simulink model "nn_fuel_control_6_20"  (R2021a)
settings: Solver=ode15s  StartTime=0.0  StopTime=T  MaxStep=.01  RelTol=1e-3
undefined symbols (not defined in the file): AF_sensor_tol, fault_time, fuel_inj_tol, kappa_tol, MAF_sensor_tol, pump_tol, tau_ww_tol
libraries: neural x128
(part 2 of 6)

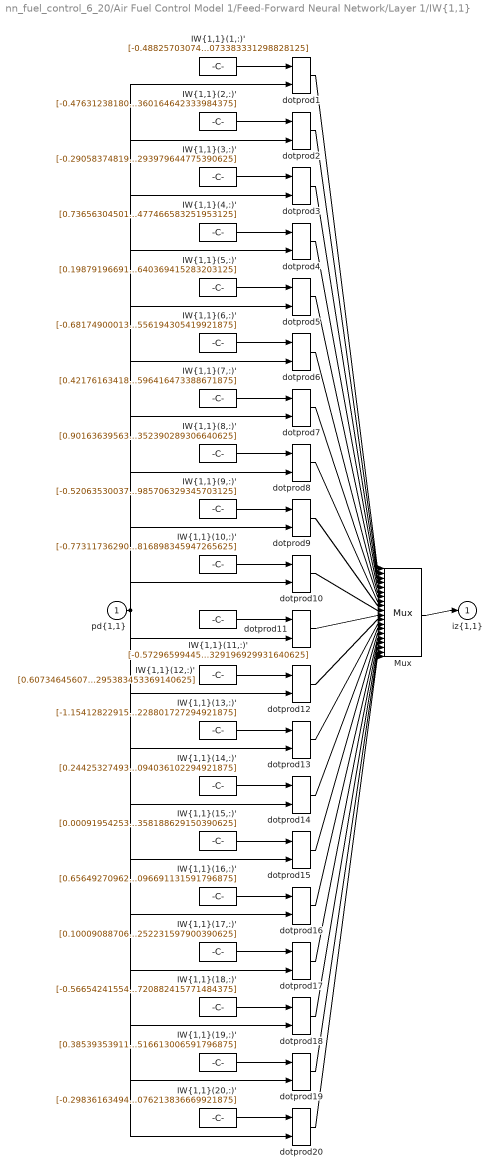
== system nn_fuel_control_6_20/Air Fuel Control Model 1/Feed-Forward Neural Network/Layer 1/IW{1,1} ==
  "pd{1,1}" : Inport  PortDimensions=4
      mask Display: e = 0.06;c1 = [120 230 180]/255;c2 = ([120 230 180]+0)/(256+128);c3 = ([120 230 180]+128)/(256+128);patch([0 1 1 0],[0 0 1 1],c1);patch([0 1 1 1-e 1-e 0+e],[0 0 1 1-e 0+e 0+e],c2);patch([0 0 1 1-e 0+e 0+e],[0 1 1 1-e 1-e 0+e],c3);plot([0 1 1 0 0],[0 0 1 1 0]);
  "IW{1,1}(1,:)'" : Constant  Value=[-0.48825703074007853476956597660318948328495025634765625;-0.571856754184941085128457416431047022342681884765625;-0.40434581347511555637908031712868250906467437744140625;0.33801748115781393710932434260030277073383331298828125]
      mask Display: e = 0.06;c1 = [120 150 230]/255;c2 = ([120 150 230]+0)/383;c3 = ([120 150 230]+128)/383;patch([0 1 1 0],[0 0 1 1],c1);patch([0 1 1 1-e 1-e 0+e],[0 0 1 1-e 0+e 0+e],c2);patch([0 0 1 1-e 0+e 0+e],[0 1 1 1-e 1-e 0+e],c3);plot([0 1 1 0 0],[0 0 1 1 0]);disp('Weights');
  "IW{1,1}(10,:)'" : Constant  Value=[-0.7731173629085674736671762730111368000507354736328125;0.2005059506174451389171053961035795509815216064453125;0.1626130441440647445006106863729655742645263671875;0.1745533013814315470568772070691920816898345947265625]
      mask Display: e = 0.06;c1 = [120 150 230]/255;c2 = ([120 150 230]+0)/383;c3 = ([120 150 230]+128)/383;patch([0 1 1 0],[0 0 1 1],c1);patch([0 1 1 1-e 1-e 0+e],[0 0 1 1-e 0+e 0+e],c2);patch([0 0 1 1-e 0+e 0+e],[0 1 1 1-e 1-e 0+e],c3);plot([0 1 1 0 0],[0 0 1 1 0]);disp('Weights');
  "IW{1,1}(11,:)'" : Constant  Value=[-0.57296599445932028249472978131962008774280548095703125;0.486466690002032298156819933865335769951343536376953125;0.59005984322004934039540557932923547923564910888671875;0.478764443667865580156473015449591912329196929931640625]
      mask Display: e = 0.06;c1 = [120 150 230]/255;c2 = ([120 150 230]+0)/383;c3 = ([120 150 230]+128)/383;patch([0 1 1 0],[0 0 1 1],c1);patch([0 1 1 1-e 1-e 0+e],[0 0 1 1-e 0+e 0+e],c2);patch([0 0 1 1-e 0+e 0+e],[0 1 1 1-e 1-e 0+e],c3);plot([0 1 1 0 0],[0 0 1 1 0]);disp('Weights');
  "IW{1,1}(12,:)'" : Constant  Value=[0.60734645607013415524733090933295898139476776123046875;-0.56727561458132924609998326559434644877910614013671875;-0.3464328462213754900034246020368300378322601318359375;0.01188492491926852225037070098778713145293295383453369140625]
      mask Display: e = 0.06;c1 = [120 150 230]/255;c2 = ([120 150 230]+0)/383;c3 = ([120 150 230]+128)/383;patch([0 1 1 0],[0 0 1 1],c1);patch([0 1 1 1-e 1-e 0+e],[0 0 1 1-e 0+e 0+e],c2);patch([0 0 1 1-e 0+e 0+e],[0 1 1 1-e 1-e 0+e],c3);plot([0 1 1 0 0],[0 0 1 1 0]);disp('Weights');
  "IW{1,1}(13,:)'" : Constant  Value=[-1.1541282291561423267722830132697708904743194580078125;-0.367041931636175267072985661798156797885894775390625;0.00571687256956400491336722780033596791326999664306640625;-1.1769488295019250312378744638408534228801727294921875]
      mask Display: e = 0.06;c1 = [120 150 230]/255;c2 = ([120 150 230]+0)/383;c3 = ([120 150 230]+128)/383;patch([0 1 1 0],[0 0 1 1],c1);patch([0 1 1 1-e 1-e 0+e],[0 0 1 1-e 0+e 0+e],c2);patch([0 0 1 1-e 0+e 0+e],[0 1 1 1-e 1-e 0+e],c3);plot([0 1 1 0 0],[0 0 1 1 0]);disp('Weights');
  "IW{1,1}(14,:)'" : Constant  Value=[0.2442532749352764043226926560237188823521137237548828125;-1.8079559641845570627793904350255616009235382080078125;-0.84702514936941530887537510352558456361293792724609375;0.71981418547994457934890988326515071094036102294921875]
      mask Display: e = 0.06;c1 = [120 150 230]/255;c2 = ([120 150 230]+0)/383;c3 = ([120 150 230]+128)/383;patch([0 1 1 0],[0 0 1 1],c1);patch([0 1 1 1-e 1-e 0+e],[0 0 1 1-e 0+e 0+e],c2);patch([0 0 1 1-e 0+e 0+e],[0 1 1 1-e 1-e 0+e],c3);plot([0 1 1 0 0],[0 0 1 1 0]);disp('Weights');
  "IW{1,1}(15,:)'" : Constant  Value=[0.00091954253676776779267976191789557560696266591548919677734375;0.58230594094139209726535000299918465316295623779296875;-0.1812579368778876320877913030926720239222049713134765625;0.81865583686941756358379507219069637358188629150390625]
      mask Display: e = 0.06;c1 = [120 150 230]/255;c2 = ([120 150 230]+0)/383;c3 = ([120 150 230]+128)/383;patch([0 1 1 0],[0 0 1 1],c1);patch([0 1 1 1-e 1-e 0+e],[0 0 1 1-e 0+e 0+e],c2);patch([0 0 1 1-e 0+e 0+e],[0 1 1 1-e 1-e 0+e],c3);plot([0 1 1 0 0],[0 0 1 1 0]);disp('Weights');
  "IW{1,1}(16,:)'" : Constant  Value=[0.65649270962487193958878606281359679996967315673828125;-0.76315614470481663023093688025255687534809112548828125;0.301942106699343681963654262290219776332378387451171875;0.17120717116793560119702988231438212096691131591796875]
      mask Display: e = 0.06;c1 = [120 150 230]/255;c2 = ([120 150 230]+0)/383;c3 = ([120 150 230]+128)/383;patch([0 1 1 0],[0 0 1 1],c1);patch([0 1 1 1-e 1-e 0+e],[0 0 1 1-e 0+e 0+e],c2);patch([0 0 1 1-e 0+e 0+e],[0 1 1 1-e 1-e 0+e],c3);plot([0 1 1 0 0],[0 0 1 1 0]);disp('Weights');
  "IW{1,1}(17,:)'" : Constant  Value=[0.10009088706659761969230970635180710814893245697021484375;0.283349138687722490459464097511954605579376220703125;-0.33980594650471385165246829274110496044158935546875;0.0191029179120060545182813172004898660816252231597900390625]
      mask Display: e = 0.06;c1 = [120 150 230]/255;c2 = ([120 150 230]+0)/383;c3 = ([120 150 230]+128)/383;patch([0 1 1 0],[0 0 1 1],c1);patch([0 1 1 1-e 1-e 0+e],[0 0 1 1-e 0+e 0+e],c2);patch([0 0 1 1-e 0+e 0+e],[0 1 1 1-e 1-e 0+e],c3);plot([0 1 1 0 0],[0 0 1 1 0]);disp('Weights');
  "IW{1,1}(18,:)'" : Constant  Value=[-0.5665424155432698949397263277205638587474822998046875;-0.54033955185199145088148497961810790002346038818359375;0.279081720790874066029374489517067559063434600830078125;0.47911903792710874849802848984836600720882415771484375]
      mask Display: e = 0.06;c1 = [120 150 230]/255;c2 = ([120 150 230]+0)/383;c3 = ([120 150 230]+128)/383;patch([0 1 1 0],[0 0 1 1],c1);patch([0 1 1 1-e 1-e 0+e],[0 0 1 1-e 0+e 0+e],c2);patch([0 0 1 1-e 0+e 0+e],[0 1 1 1-e 1-e 0+e],c3);plot([0 1 1 0 0],[0 0 1 1 0]);disp('Weights');
  "IW{1,1}(19,:)'" : Constant  Value=[0.3853935391181619873890440430841408669948577880859375;-0.383574085589689861564011152950115501880645751953125;-0.5416431443522891076014502687030471861362457275390625;-0.981747569426136390546844268101267516613006591796875]
      mask Display: e = 0.06;c1 = [120 150 230]/255;c2 = ([120 150 230]+0)/383;c3 = ([120 150 230]+128)/383;patch([0 1 1 0],[0 0 1 1],c1);patch([0 1 1 1-e 1-e 0+e],[0 0 1 1-e 0+e 0+e],c2);patch([0 0 1 1-e 0+e 0+e],[0 1 1 1-e 1-e 0+e],c3);plot([0 1 1 0 0],[0 0 1 1 0]);disp('Weights');
  "IW{1,1}(2,:)'" : Constant  Value=[-0.4763123818029502132276320480741560459136962890625;-0.3624779463226779352424955504829995334148406982421875;0.548920167863276020625562523491680622100830078125;-0.9809602571508406754219322465360164642333984375]
      mask Display: e = 0.06;c1 = [120 150 230]/255;c2 = ([120 150 230]+0)/383;c3 = ([120 150 230]+128)/383;patch([0 1 1 0],[0 0 1 1],c1);patch([0 1 1 1-e 1-e 0+e],[0 0 1 1-e 0+e 0+e],c2);patch([0 0 1 1-e 0+e 0+e],[0 1 1 1-e 1-e 0+e],c3);plot([0 1 1 0 0],[0 0 1 1 0]);disp('Weights');
  "IW{1,1}(20,:)'" : Constant  Value=[-0.2983616349407973711294062013621442019939422607421875;-0.904882675555897630914614637731574475765228271484375;0.3663740946078786198114585204166360199451446533203125;-0.377532327383313326407687782193534076213836669921875]
      mask Display: e = 0.06;c1 = [120 150 230]/255;c2 = ([120 150 230]+0)/383;c3 = ([120 150 230]+128)/383;patch([0 1 1 0],[0 0 1 1],c1);patch([0 1 1 1-e 1-e 0+e],[0 0 1 1-e 0+e 0+e],c2);patch([0 0 1 1-e 0+e 0+e],[0 1 1 1-e 1-e 0+e],c3);plot([0 1 1 0 0],[0 0 1 1 0]);disp('Weights');
  "IW{1,1}(3,:)'" : Constant  Value=[-0.2905837481960433787975262021063826978206634521484375;0.109981844822967911312616706709377467632293701171875;0.455515839932046084914674111132626421749591827392578125;-0.8132927338045536913568867021240293979644775390625]
      mask Display: e = 0.06;c1 = [120 150 230]/255;c2 = ([120 150 230]+0)/383;c3 = ([120 150 230]+128)/383;patch([0 1 1 0],[0 0 1 1],c1);patch([0 1 1 1-e 1-e 0+e],[0 0 1 1-e 0+e 0+e],c2);patch([0 0 1 1-e 0+e 0+e],[0 1 1 1-e 1-e 0+e],c3);plot([0 1 1 0 0],[0 0 1 1 0]);disp('Weights');
  "IW{1,1}(4,:)'" : Constant  Value=[0.73656304501564962006199266397743485867977142333984375;-3.144535832691242038805512493127025663852691650390625;-1.0375718682022092576033855948480777442455291748046875;0.64654475977152092713851061489549465477466583251953125]
      mask Display: e = 0.06;c1 = [120 150 230]/255;c2 = ([120 150 230]+0)/383;c3 = ([120 150 230]+128)/383;patch([0 1 1 0],[0 0 1 1],c1);patch([0 1 1 1-e 1-e 0+e],[0 0 1 1-e 0+e 0+e],c2);patch([0 0 1 1-e 0+e 0+e],[0 1 1 1-e 1-e 0+e],c3);plot([0 1 1 0 0],[0 0 1 1 0]);disp('Weights');
  "IW{1,1}(5,:)'" : Constant  Value=[0.198791966914059037296880205758498050272464752197265625;-0.1633450522665338133787571450739051215350627899169921875;0.42744201772333045852292343624867498874664306640625;0.256072707330624649291195282785338349640369415283203125]
      mask Display: e = 0.06;c1 = [120 150 230]/255;c2 = ([120 150 230]+0)/383;c3 = ([120 150 230]+128)/383;patch([0 1 1 0],[0 0 1 1],c1);patch([0 1 1 1-e 1-e 0+e],[0 0 1 1-e 0+e 0+e],c2);patch([0 0 1 1-e 0+e 0+e],[0 1 1 1-e 1-e 0+e],c3);plot([0 1 1 0 0],[0 0 1 1 0]);disp('Weights');
  "IW{1,1}(6,:)'" : Constant  Value=[-0.68174900013601558157461113296449184417724609375;-0.143660359213997057548084512745845131576061248779296875;-0.017244855890485570604209186740263248793780803680419921875;-0.59564977304797117607648715420509688556194305419921875]
      mask Display: e = 0.06;c1 = [120 150 230]/255;c2 = ([120 150 230]+0)/383;c3 = ([120 150 230]+128)/383;patch([0 1 1 0],[0 0 1 1],c1);patch([0 1 1 1-e 1-e 0+e],[0 0 1 1-e 0+e 0+e],c2);patch([0 0 1 1-e 0+e 0+e],[0 1 1 1-e 1-e 0+e],c3);plot([0 1 1 0 0],[0 0 1 1 0]);disp('Weights');
  "IW{1,1}(7,:)'" : Constant  Value=[0.4217616341804173440976910569588653743267059326171875;0.268686773032350334489137821947224438190460205078125;-0.7596642819355239328871221005101688206195831298828125;0.1140485715139589739663961154292337596416473388671875]
      mask Display: e = 0.06;c1 = [120 150 230]/255;c2 = ([120 150 230]+0)/383;c3 = ([120 150 230]+128)/383;patch([0 1 1 0],[0 0 1 1],c1);patch([0 1 1 1-e 1-e 0+e],[0 0 1 1-e 0+e 0+e],c2);patch([0 0 1 1-e 0+e 0+e],[0 1 1 1-e 1-e 0+e],c3);plot([0 1 1 0 0],[0 0 1 1 0]);disp('Weights');
  "IW{1,1}(8,:)'" : Constant  Value=[0.9016363956360040621262896820553578436374664306640625;0.357548177780251108526243797314236871898174285888671875;0.55252323002836389864711463815183378756046295166015625;-0.060258972495788688805706811990603455342352390289306640625]
      mask Display: e = 0.06;c1 = [120 150 230]/255;c2 = ([120 150 230]+0)/383;c3 = ([120 150 230]+128)/383;patch([0 1 1 0],[0 0 1 1],c1);patch([0 1 1 1-e 1-e 0+e],[0 0 1 1-e 0+e 0+e],c2);patch([0 0 1 1-e 0+e 0+e],[0 1 1 1-e 1-e 0+e],c3);plot([0 1 1 0 0],[0 0 1 1 0]);disp('Weights');
  "IW{1,1}(9,:)'" : Constant  Value=[-0.52063530037897998159479584501241333782672882080078125;0.81677809495395992112065641777007840573787689208984375;-0.95310858934972031430987726707826368510723114013671875;0.325348652875194599420893837304902262985706329345703125]
      mask Display: e = 0.06;c1 = [120 150 230]/255;c2 = ([120 150 230]+0)/383;c3 = ([120 150 230]+128)/383;patch([0 1 1 0],[0 0 1 1],c1);patch([0 1 1 1-e 1-e 0+e],[0 0 1 1-e 0+e 0+e],c2);patch([0 0 1 1-e 0+e 0+e],[0 1 1 1-e 1-e 0+e],c3);plot([0 1 1 0 0],[0 0 1 1 0]);disp('Weights');
  Mux : Mux  Inputs=20
      mask Display: e = 0.06;c1 = [120 150 230]/255;c2 = ([120 150 230]+0)/383;c3 = ([120 150 230]+128)/383;patch([0 1 1 0],[0 0 1 1],c1);patch([0 1 1 1-e 1-e 0+e],[0 0 1 1-e 0+e 0+e],c2);patch([0 0 1 1-e 0+e 0+e],[0 1 1 1-e 1-e 0+e],c3);plot([0 1 1 0 0],[0 0 1 1 0]);disp('Mux');
  dotprod{1..20} (20 alike) : neural/Weight Functions/dotprod
  "iz{1,1}" : Outport
      mask Display: e = 0.06;c1 = [120 230 180]/255;c2 = ([120 230 180]+0)/(256+128);c3 = ([120 230 180]+128)/(256+128);patch([0 1 1 0],[0 0 1 1],c1);patch([0 1 1 1-e 1-e 0+e],[0 0 1 1-e 0+e 0+e],c2);patch([0 0 1 1-e 0+e 0+e],[0 1 1 1-e 1-e 0+e],c3);plot([0 1 1 0 0],[0 0 1 1 0]);
  wires:
  "IW{1,1}(1,:)'"/1 -> dotprod1/1
  "pd{1,1}"/1 -> dotprod1/2, dotprod2/2, dotprod3/2, dotprod4/2, dotprod5/2, dotprod6/2, dotprod7/2, dotprod8/2, dotprod9/2, dotprod10/2, dotprod11/2, dotprod12/2, dotprod13/2, dotprod14/2, dotprod15/2, dotprod16/2, dotprod17/2, dotprod18/2, dotprod19/2, dotprod20/2
  dotprod1/1 -> Mux/1
  "IW{1,1}(2,:)'"/1 -> dotprod2/1
  dotprod2/1 -> Mux/2
  "IW{1,1}(3,:)'"/1 -> dotprod3/1
  dotprod3/1 -> Mux/3
  "IW{1,1}(4,:)'"/1 -> dotprod4/1
  dotprod4/1 -> Mux/4
  "IW{1,1}(5,:)'"/1 -> dotprod5/1
  dotprod5/1 -> Mux/5
  "IW{1,1}(6,:)'"/1 -> dotprod6/1
  dotprod6/1 -> Mux/6
  "IW{1,1}(7,:)'"/1 -> dotprod7/1
  dotprod7/1 -> Mux/7
  "IW{1,1}(8,:)'"/1 -> dotprod8/1
  dotprod8/1 -> Mux/8
  "IW{1,1}(9,:)'"/1 -> dotprod9/1
  dotprod9/1 -> Mux/9
  "IW{1,1}(10,:)'"/1 -> dotprod10/1
  dotprod10/1 -> Mux/10
  "IW{1,1}(11,:)'"/1 -> dotprod11/1
  dotprod11/1 -> Mux/11
  "IW{1,1}(12,:)'"/1 -> dotprod12/1
  dotprod12/1 -> Mux/12
  "IW{1,1}(13,:)'"/1 -> dotprod13/1
  dotprod13/1 -> Mux/13
  "IW{1,1}(14,:)'"/1 -> dotprod14/1
  dotprod14/1 -> Mux/14
  "IW{1,1}(15,:)'"/1 -> dotprod15/1
  dotprod15/1 -> Mux/15
  "IW{1,1}(16,:)'"/1 -> dotprod16/1
  dotprod16/1 -> Mux/16
  "IW{1,1}(17,:)'"/1 -> dotprod17/1
  dotprod17/1 -> Mux/17
  "IW{1,1}(18,:)'"/1 -> dotprod18/1
  dotprod18/1 -> Mux/18
  "IW{1,1}(19,:)'"/1 -> dotprod19/1
  dotprod19/1 -> Mux/19
  "IW{1,1}(20,:)'"/1 -> dotprod20/1
  dotprod20/1 -> Mux/20
  Mux/1 -> "iz{1,1}"/1

== system nn_fuel_control_6_20/Air Fuel Control Model 1/Feed-Forward Neural Network/Layer 2/Delays 1 ==
  "p{2}" : Inport  PortDimensions=20
      mask Display: e = 0.06;c1 = [120 230 180]/255;c2 = ([120 230 180]+0)/(256+128);c3 = ([120 230 180]+128)/(256+128);patch([0 1 1 0],[0 0 1 1],c1);patch([0 1 1 1-e 1-e 0+e],[0 0 1 1-e 0+e 0+e],c2);patch([0 0 1 1-e 0+e 0+e],[0 1 1 1-e 1-e 0+e],c3);plot([0 1 1 0 0],[0 0 1 1 0]);
  mux : Mux  Inputs=1
      mask Display: e = 0.06;c1 = [120 150 230]/255;c2 = ([120 150 230]+0)/383;c3 = ([120 150 230]+128)/383;patch([0 1 1 0],[0 0 1 1],c1);patch([0 1 1 1-e 1-e 0+e],[0 0 1 1-e 0+e 0+e],c2);patch([0 0 1 1-e 0+e 0+e],[0 1 1 1-e 1-e 0+e],c3);plot([0 1 1 0 0],[0 0 1 1 0]);disp('Mux')
  "pd{2,1}" : Outport
      mask Display: e = 0.06;c1 = [120 230 180]/255;c2 = ([120 230 180]+0)/(256+128);c3 = ([120 230 180]+128)/(256+128);patch([0 1 1 0],[0 0 1 1],c1);patch([0 1 1 1-e 1-e 0+e],[0 0 1 1-e 0+e 0+e],c2);patch([0 0 1 1-e 0+e 0+e],[0 1 1 1-e 1-e 0+e],c3);plot([0 1 1 0 0],[0 0 1 1 0]);
  wires:
  "p{2}"/1 -> mux/1
  mux/1 -> "pd{2,1}"/1

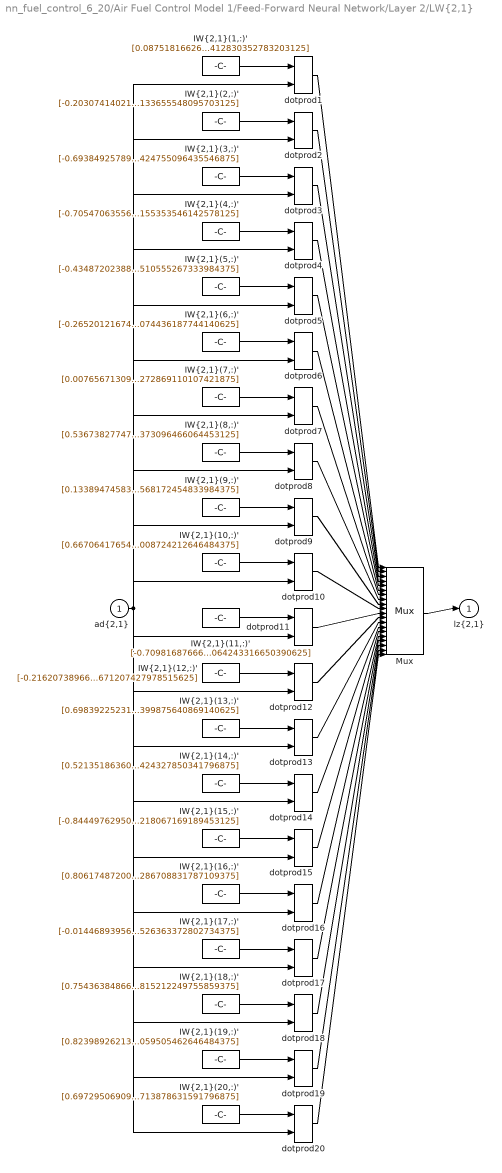
== system nn_fuel_control_6_20/Air Fuel Control Model 1/Feed-Forward Neural Network/Layer 2/LW{2,1} ==
  "ad{2,1}" : Inport  PortDimensions=20
      mask Display: e = 0.06;c1 = [120 230 180]/255;c2 = ([120 230 180]+0)/(256+128);c3 = ([120 230 180]+128)/(256+128);patch([0 1 1 0],[0 0 1 1],c1);patch([0 1 1 1-e 1-e 0+e],[0 0 1 1-e 0+e 0+e],c2);patch([0 0 1 1-e 0+e 0+e],[0 1 1 1-e 1-e 0+e],c3);plot([0 1 1 0 0],[0 0 1 1 0]);
  "IW{2,1}(1,:)'" : Constant  Value=[0.0875181662665719117821794270639657042920589447021484375;0.921321050546581421514247267623431980609893798828125;-0.1717118974253677432528775170794688165187835693359375;-0.68304825916014200171133552430546842515468597412109375;0.452339285545516556208411884654196910560131072998046875;-0.04529182730159657388480098916261340491473674774169921875;-0.9709510342483935740887091014883480966091156005859375;0.020509492560360172153099966863010195083916187286376953125;0.78509599817010677913486915713292546570301055908203125;-0.4830724448255014902287030054139904677867889404296875;0.89266777388446183483239337874692864716053009033203125;0.042941053928391655081231448320977506227791309356689453125;-0.1415144968584703122349566228876938112080097198486328125;-1.2230150910133141817226487546577118337154388427734375;0.1333293552699185424703642866006703115999698638916015625;-0.9177651014595056278011497852276079356670379638671875;-0.1228244578666999320404329409939236938953399658203125;0.5867901928731706906461340622627176344394683837890625;0.63198665556140465326961930259130895137786865234375;0.8997269280854862660845583377522416412830352783203125]
      mask Display: e = 0.06;c1 = [120 150 230]/255;c2 = ([120 150 230]+0)/383;c3 = ([120 150 230]+128)/383;patch([0 1 1 0],[0 0 1 1],c1);patch([0 1 1 1-e 1-e 0+e],[0 0 1 1-e 0+e 0+e],c2);patch([0 0 1 1-e 0+e 0+e],[0 1 1 1-e 1-e 0+e],c3);plot([0 1 1 0 0],[0 0 1 1 0]);disp('weights');
  "IW{2,1}(10,:)'" : Constant  Value=[0.6670641765450044946561547476449050009250640869140625;-0.514079267728301037010396612458862364292144775390625;0.4412099253120829178698159012128598988056182861328125;0.365585408566961145293561230573686771094799041748046875;-0.101844567281333564512380007727188058197498321533203125;1.0234943592269705181507788438466377556324005126953125;-0.2964378932206355177214618379366584122180938720703125;0.89165504879323720377470863240887410938739776611328125;0.00071741415381627871017400366326910443603992462158203125;-0.35129661907085729666277984506450593471527099609375;-0.08630387658328413091890496389169129543006420135498046875;0.73285931796011050121109065003111027181148529052734375;0.9141116517940217622850695988745428621768951416015625;-0.5898122749869834091640541373635642230510711669921875;0.5581383460192237411234827959560789167881011962890625;-0.391394620189690234379753519533551298081874847412109375;-0.56609108316777534408714700475684367120265960693359375;-0.78857350176913987294113894677138887345790863037109375;-0.1110936003246558723134285173728130757808685302734375;0.144677769719792959079995853244327008724212646484375]
      mask Display: e = 0.06;c1 = [120 150 230]/255;c2 = ([120 150 230]+0)/383;c3 = ([120 150 230]+128)/383;patch([0 1 1 0],[0 0 1 1],c1);patch([0 1 1 1-e 1-e 0+e],[0 0 1 1-e 0+e 0+e],c2);patch([0 0 1 1-e 0+e 0+e],[0 1 1 1-e 1-e 0+e],c3);plot([0 1 1 0 0],[0 0 1 1 0]);disp('weights');
  "IW{2,1}(11,:)'" : Constant  Value=[-0.709816876661096163303454886772669851779937744140625;-0.3444212300521931613417336848215200006961822509765625;0.9832500828514560975435188083793036639690399169921875;-0.43613745027057049252761089519481174647808074951171875;-0.55211644185470853951613889876171015202999114990234375;-0.7575041344288002687079597308184020221233367919921875;-0.2847945211821218958192503123427741229534149169921875;-0.07355592846682361407584238577328505925834178924560546875;0.634284151179720812052664768998511135578155517578125;-0.442299985847484311562993752886541187763214111328125;0.2745419011869854042373617630801163613796234130859375;-0.78469757805809281503428564974456094205379486083984375;-0.9078653485353538332702783009153790771961212158203125;0.08518212744205312658696271910230279900133609771728515625;-0.63299556814274715588197750548715703189373016357421875;0.94372659672676306730210171735961921513080596923828125;-0.86235896127647826414630571889574639499187469482421875;-0.36254626539261336493069620701135136187076568603515625;-0.9987256219878009044776945302146486937999725341796875;0.56472885556065310908024912350811064243316650390625]
      mask Display: e = 0.06;c1 = [120 150 230]/255;c2 = ([120 150 230]+0)/383;c3 = ([120 150 230]+128)/383;patch([0 1 1 0],[0 0 1 1],c1);patch([0 1 1 1-e 1-e 0+e],[0 0 1 1-e 0+e 0+e],c2);patch([0 0 1 1-e 0+e 0+e],[0 1 1 1-e 1-e 0+e],c3);plot([0 1 1 0 0],[0 0 1 1 0]);disp('weights');
  "IW{2,1}(12,:)'" : Constant  Value=[-0.2162073896661820260334252452594228088855743408203125;-0.761704303295197338030675382469780743122100830078125;0.124054668622003816391696773280273191630840301513671875;0.0666422255806751184792346975882537662982940673828125;-0.1018576594486159392349833296975702978670597076416015625;-0.7633396770781526452509524460765533149242401123046875;0.80878320521564450729101736214943230152130126953125;0.9107228523006707376907797879539430141448974609375;0.68803687900472876304291958149406127631664276123046875;-0.673404946456113151498357183299958705902099609375;0.02618620323267932537003588322477298788726329803466796875;-0.1434357633318594504867604655373725108802318572998046875;-0.2081794769619056684195612660914775915443897247314453125;0.82206885550436370468929681010195054113864898681640625;1.3395412792208656327375138062052428722381591796875;0.5779458927466978312992296196171082556247711181640625;-0.026880949945973141301802655789288110099732875823974609375;0.850129415928704279536987087340094149112701416015625;0.761799842289866635525186211452819406986236572265625;-0.7519111742583659552252584035159088671207427978515625]
      mask Display: e = 0.06;c1 = [120 150 230]/255;c2 = ([120 150 230]+0)/383;c3 = ([120 150 230]+128)/383;patch([0 1 1 0],[0 0 1 1],c1);patch([0 1 1 1-e 1-e 0+e],[0 0 1 1-e 0+e 0+e],c2);patch([0 0 1 1-e 0+e 0+e],[0 1 1 1-e 1-e 0+e],c3);plot([0 1 1 0 0],[0 0 1 1 0]);disp('weights');
  "IW{2,1}(13,:)'" : Constant  Value=[0.698392252312435513061927849776111543178558349609375;0.2006250289554845078754397036391310393810272216796875;0.8979808453752837760220018026302568614482879638671875;0.13058294946861292995521353077492676675319671630859375;0.6337289839007096414746911250404082238674163818359375;-0.4606636658097738035166912595741450786590576171875;0.58270529187201436371879026410169899463653564453125;-0.334455647345431150707639744723564945161342620849609375;0.432404381050130848240797831749659962952136993408203125;-0.5325686929910187217274142312817275524139404296875;-1.071395629971807039737541344948112964630126953125;0.01201015671242645910243851403720327652990818023681640625;-0.86364459893233791465405602139071561396121978759765625;0.44599042299617075446604985700105316936969757080078125;0.387361224848535135034666154751903377473354339599609375;0.5979970960929346102119552597287110984325408935546875;0.0432920224562478583862912273616530001163482666015625;0.347379189552733003143458745398675091564655303955078125;-0.810953983836439906696114121587015688419342041015625;0.123159835575779030847343165078200399875640869140625]
      mask Display: e = 0.06;c1 = [120 150 230]/255;c2 = ([120 150 230]+0)/383;c3 = ([120 150 230]+128)/383;patch([0 1 1 0],[0 0 1 1],c1);patch([0 1 1 1-e 1-e 0+e],[0 0 1 1-e 0+e 0+e],c2);patch([0 0 1 1-e 0+e 0+e],[0 1 1 1-e 1-e 0+e],c3);plot([0 1 1 0 0],[0 0 1 1 0]);disp('weights');
  "IW{2,1}(14,:)'" : Constant  Value=[0.52135186360587326692694887242396362125873565673828125;0.76681461221118496496274019591510295867919921875;0.182440316929996904082855735396151430904865264892578125;-0.667185236925864177948142241802997887134552001953125;0.018186640242936778777416151342549710534512996673583984375;-0.4881029077366729751474849763326346874237060546875;0.979122095289337579515631659887731075286865234375;0.381131888419126763078992325972649268805980682373046875;0.01950508251932532577388457184497383423149585723876953125;0.573841738425475256235586130060255527496337890625;0.77623766667199578517255531551199965178966522216796875;-0.74760112641349130147006007973686791956424713134765625;0.39764422671061583347551504630246199667453765869140625;0.594832565933728130147528645466081798076629638671875;-0.527690451082258871196017935290001332759857177734375;0.036548739067653678025404673235243535600602626800537109375;0.7462124283112026024156193670933134853839874267578125;0.197709760210736884555871029078844003379344940185546875;0.0637598096026212868281390910851769149303436279296875;-0.005816547577797148704803475993685424327850341796875]
      mask Display: e = 0.06;c1 = [120 150 230]/255;c2 = ([120 150 230]+0)/383;c3 = ([120 150 230]+128)/383;patch([0 1 1 0],[0 0 1 1],c1);patch([0 1 1 1-e 1-e 0+e],[0 0 1 1-e 0+e 0+e],c2);patch([0 0 1 1-e 0+e 0+e],[0 1 1 1-e 1-e 0+e],c3);plot([0 1 1 0 0],[0 0 1 1 0]);disp('weights');
  "IW{2,1}(15,:)'" : Constant  Value=[-0.844497629509766145616822541342116892337799072265625;-0.376646781418800369323207632987760007381439208984375;-0.2496606881963896740206365620906581170856952667236328125;0.156946624742526907869688557184417732059955596923828125;0.3628703975687013194573182772728614509105682373046875;0.739224653174116230758272649836726486682891845703125;-0.8475195754241118262228837920702062547206878662109375;-0.467202132042335016581802165092085488140583038330078125;0.53251643923307734329597451505833305418491363525390625;0.453277783012928647821127015049569308757781982421875;-0.84634472740554567149473541576298885047435760498046875;-0.16446613172345669884322205689386464655399322509765625;-0.6832508944670252493125417458941228687763214111328125;0.35031433065206230015320443271775729954242706298828125;0.59911140187267453161013008866575546562671661376953125;0.037948459690654266773801595036275102756917476654052734375;0.83051324880117405324853052661637775599956512451171875;-0.8633126310479466436476059243432246148586273193359375;0.384422756775311125210237150895409286022186279296875;-0.2735283149473748398605721376952715218067169189453125]
      mask Display: e = 0.06;c1 = [120 150 230]/255;c2 = ([120 150 230]+0)/383;c3 = ([120 150 230]+128)/383;patch([0 1 1 0],[0 0 1 1],c1);patch([0 1 1 1-e 1-e 0+e],[0 0 1 1-e 0+e 0+e],c2);patch([0 0 1 1-e 0+e 0+e],[0 1 1 1-e 1-e 0+e],c3);plot([0 1 1 0 0],[0 0 1 1 0]);disp('weights');
  "IW{2,1}(16,:)'" : Constant  Value=[0.8061748720068087070700357799069024622440338134765625;0.6763532480856941919711289301631040871143341064453125;0.60268412899608225785641479887999594211578369140625;-0.76203207642208514727144574862904846668243408203125;0.496598615700733325706295318013872019946575164794921875;0.2256072642750229506614090269067673943936824798583984375;0.5279125451586981210283511245506815612316131591796875;0.12499657115886254887815454139854409731924533843994140625;0.51111045401448651492870567381032742559909820556640625;-0.626459610685625722936720194411464035511016845703125;-0.01034574018027341335557167667502653785049915313720703125;-0.272728270147501616893492837334633804857730865478515625;-0.32125403341735070394946660599089227616786956787109375;0.280656809280696639685714899314916692674160003662109375;-0.427629322977498615987457242226810194551944732666015625;-0.7257714231649823322101156009011901915073394775390625;0.1307553822847522528860508828074671328067779541015625;-0.6537562916574024551863431042875163257122039794921875;-0.94115208881642065108508177218027412891387939453125;0.5900674660015672312596279880381189286708831787109375]
      mask Display: e = 0.06;c1 = [120 150 230]/255;c2 = ([120 150 230]+0)/383;c3 = ([120 150 230]+128)/383;patch([0 1 1 0],[0 0 1 1],c1);patch([0 1 1 1-e 1-e 0+e],[0 0 1 1-e 0+e 0+e],c2);patch([0 0 1 1-e 0+e 0+e],[0 1 1 1-e 1-e 0+e],c3);plot([0 1 1 0 0],[0 0 1 1 0]);disp('weights');
  "IW{2,1}(17,:)'" : Constant  Value=[-0.014468939568756000735305633497773669660091400146484375;0.8752557726079090993920317487209104001522064208984375;-0.705229439017080128593306653783656656742095947265625;1.039642515692225099854795189457945525646209716796875;0.299769597407585963733112066620378755033016204833984375;-0.057230890442454496191970747531740926206111907958984375;-0.940801928295217582132181632914580404758453369140625;-0.37262187634401400249117841667612083256244659423828125;0.004182310526150700979997054673731327056884765625;-0.6660681331177842334767547072260640561580657958984375;0.9565564952174001600582187165855430066585540771484375;-1.041982357923853630410349069279618561267852783203125;-0.6285797327742190798716137578594498336315155029296875;-0.492423136017870632930026886242558248341083526611328125;-0.492219218043910389237538538509397767484188079833984375;0.19331991296376160871517413397668860852718353271484375;0.71220735263215961818872301591909490525722503662109375;-0.34626382952495127209857628258760087192058563232421875;-0.92328728685487693184086310793645679950714111328125;0.2984772211431356847555207423283718526363372802734375]
      mask Display: e = 0.06;c1 = [120 150 230]/255;c2 = ([120 150 230]+0)/383;c3 = ([120 150 230]+128)/383;patch([0 1 1 0],[0 0 1 1],c1);patch([0 1 1 1-e 1-e 0+e],[0 0 1 1-e 0+e 0+e],c2);patch([0 0 1 1-e 0+e 0+e],[0 1 1 1-e 1-e 0+e],c3);plot([0 1 1 0 0],[0 0 1 1 0]);disp('weights');
  "IW{2,1}(18,:)'" : Constant  Value=[0.754363848668714975786997456452809274196624755859375;-0.33817682986599351124823442660272121429443359375;-1.008250270567170314706118006142787635326385498046875;-0.55224907394053557307955770738772116601467132568359375;-0.281351354763303529438189798383973538875579833984375;-0.840581794384416269849680247716605663299560546875;0.4523444464019552579969740691012702882289886474609375;-0.333482901350699523224108133945264853537082672119140625;0.85487628829904183103138848309754393994808197021484375;0.4403315907079525803879960221820510923862457275390625;-0.235251556735013689358737565271439962089061737060546875;0.53159329250477027617449721219600178301334381103515625;0.08523816875219518418571595930188777856528759002685546875;-0.50649169757445677841900533167063258588314056396484375;-0.104206419704382102775497287439065985381603240966796875;-0.55791917845603478109950401631067506968975067138671875;-0.0024601298984177383429028385108949805726297199726104736328125;0.83816611825571218918895510796573944389820098876953125;-0.603585972480569665776783949695527553558349609375;-0.8117297181718965415342381675145588815212249755859375]
      mask Display: e = 0.06;c1 = [120 150 230]/255;c2 = ([120 150 230]+0)/383;c3 = ([120 150 230]+128)/383;patch([0 1 1 0],[0 0 1 1],c1);patch([0 1 1 1-e 1-e 0+e],[0 0 1 1-e 0+e 0+e],c2);patch([0 0 1 1-e 0+e 0+e],[0 1 1 1-e 1-e 0+e],c3);plot([0 1 1 0 0],[0 0 1 1 0]);disp('weights');
  "IW{2,1}(19,:)'" : Constant  Value=[0.82398926213628598258509327934007160365581512451171875;0.9706899928354906226246612277464009821414947509765625;-0.68273943196607256300723065578495152294635772705078125;0.85150184240932336177110073549556545913219451904296875;-0.324276427260644706240810819508624263107776641845703125;-0.69999807798562263538855177102959714829921722412109375;-0.9834166185722812425495931165642105042934417724609375;0.5470030035637536425241478355019353330135345458984375;0.1589089829575216494816913836984895169734954833984375;-0.4303291556114314797554243341437540948390960693359375;-0.048500710859881390746295437566004693508148193359375;-0.50752200936306468559422455655294470489025115966796875;0.16361052925127506085800632718019187450408935546875;0.3919662601746594088325537086348049342632293701171875;1.5163554199094428920346899758442305028438568115234375;0.5119245704773167648937715057400055229663848876953125;-0.59435242351819106421118021899019367992877960205078125;1.0941868596873287611259684126707725226879119873046875;-0.184505008591826946684477661619894206523895263671875;0.4116140345428094260427087647258304059505462646484375]
      mask Display: e = 0.06;c1 = [120 150 230]/255;c2 = ([120 150 230]+0)/383;c3 = ([120 150 230]+128)/383;patch([0 1 1 0],[0 0 1 1],c1);patch([0 1 1 1-e 1-e 0+e],[0 0 1 1-e 0+e 0+e],c2);patch([0 0 1 1-e 0+e 0+e],[0 1 1 1-e 1-e 0+e],c3);plot([0 1 1 0 0],[0 0 1 1 0]);disp('weights');
  "IW{2,1}(2,:)'" : Constant  Value=[-0.203074140213432008383875881918356753885746002197265625;0.9062552814720932214953563743620179593563079833984375;0.1358198719456416292405975809742812998592853546142578125;0.6978270880328205638676308808499015867710113525390625;-0.12410640302124380240922363327626953832805156707763671875;0.70799812299052700126367199118249118328094482421875;-0.93779823626681935166971015860326588153839111328125;0.70607406406204031856788105869782157242298126220703125;-0.85243082610277454147507114612380973994731903076171875;0.6658980189558254547677051959908567368984222412109375;-0.449880727751481523934984352308674715459346771240234375;-0.1940077962190318860979942883204785175621509552001953125;0.54334821753757645002025356006924994289875030517578125;-0.57993449722908263499476788638276048004627227783203125;-0.00857207628564853052477445771728525869548320770263671875;-0.484089708841168586683778585211257450282573699951171875;0.81777236141269626923389068906544707715511322021484375;-1.067671049172129738025205369922332465648651123046875;0.3915083326027610777231302563450299203395843505859375;-0.80942485371073491506876962375827133655548095703125]
      mask Display: e = 0.06;c1 = [120 150 230]/255;c2 = ([120 150 230]+0)/383;c3 = ([120 150 230]+128)/383;patch([0 1 1 0],[0 0 1 1],c1);patch([0 1 1 1-e 1-e 0+e],[0 0 1 1-e 0+e 0+e],c2);patch([0 0 1 1-e 0+e 0+e],[0 1 1 1-e 1-e 0+e],c3);plot([0 1 1 0 0],[0 0 1 1 0]);disp('weights');
  "IW{2,1}(20,:)'" : Constant  Value=[0.697295069091591557253195787779986858367919921875;0.8672945348133171972193622423219494521617889404296875;-1.071526717931627903368507759296335279941558837890625;-1.04720814716616050787934000254608690738677978515625;-0.7161250049121843375132812070660293102264404296875;0.62612829049360119171296901185996830463409423828125;0.8565856403985814271351273418986238539218902587890625;-0.75917747491714937524420747649855911731719970703125;-0.66275538100441744315816094967885874211788177490234375;0.0703708881715510159438053960911929607391357421875;-0.177903234975636703740775601545465178787708282470703125;0.271378673216310095650527500765747390687465667724609375;0.9806891022363741772238654448301531374454498291015625;-1.1920254181944927029945802132715471088886260986328125;0.82601914724835545644765488759730942547321319580078125;0.295014101992571997623571178337442688643932342529296875;0.54185356302628850944103078290936537086963653564453125;0.280035557402768364720913041310268454253673553466796875;0.0443641830908367840180517305270768702030181884765625;-0.4828831818643368745114230478066019713878631591796875]
      mask Display: e = 0.06;c1 = [120 150 230]/255;c2 = ([120 150 230]+0)/383;c3 = ([120 150 230]+128)/383;patch([0 1 1 0],[0 0 1 1],c1);patch([0 1 1 1-e 1-e 0+e],[0 0 1 1-e 0+e 0+e],c2);patch([0 0 1 1-e 0+e 0+e],[0 1 1 1-e 1-e 0+e],c3);plot([0 1 1 0 0],[0 0 1 1 0]);disp('weights');
  "IW{2,1}(3,:)'" : Constant  Value=[-0.69384925789527596151629040832631289958953857421875;-0.4752153654035977670133661376894451677799224853515625;0.48539164049754546237380736783961765468120574951171875;-0.2096063141811837782224614556980668567121028900146484375;-0.26743830853962957672109723716857843101024627685546875;0.04183072127011232266280416070003411732614040374755859375;-0.8450531803466680980108094445313327014446258544921875;0.5226078942325076415187368183978833258152008056640625;0.7841395600703251478336142099578864872455596923828125;0.3783231528438373292289043092750944197177886962890625;0.62907281214139276759311769637861289083957672119140625;0.901737785348172504740205113193951547145843505859375;-0.56531915717772129870155595199321396648883819580078125;0.92510084619750809764582299976609647274017333984375;-0.280158395556986572483282316170516423881053924560546875;-0.472038079838744517591209159945719875395298004150390625;-0.7048478329312477530521618973580189049243927001953125;-0.63673198581909407067769279819913208484649658203125;0.9515151784234721077382346265949308872222900390625;-0.2446548509016348571520893528941087424755096435546875]
      mask Display: e = 0.06;c1 = [120 150 230]/255;c2 = ([120 150 230]+0)/383;c3 = ([120 150 230]+128)/383;patch([0 1 1 0],[0 0 1 1],c1);patch([0 1 1 1-e 1-e 0+e],[0 0 1 1-e 0+e 0+e],c2);patch([0 0 1 1-e 0+e 0+e],[0 1 1 1-e 1-e 0+e],c3);plot([0 1 1 0 0],[0 0 1 1 0]);disp('weights');
  "IW{2,1}(4,:)'" : Constant  Value=[-0.70547063556870848177737798323505558073520660400390625;0.46074665198531139509441345580853521823883056640625;0.95290877784846317322120512471883557736873626708984375;1.0492493566995306775169183310936205089092254638671875;-0.6310030076123978037827555453986860811710357666015625;-0.84697985935898356668616315801045857369899749755859375;-0.9723643975331948130502723870449699461460113525390625;0.6130920285738366004579802392981946468353271484375;-0.341786451064713669989458821873995475471019744873046875;0.3751516161106336344488454415113665163516998291015625;0.53228476256341672456784408495877869427204132080078125;0.9709600431252074503873927824315614998340606689453125;0.90513581768368667201940525046666152775287628173828125;0.38470366222370611097858272842131555080413818359375;0.411197601286168057388437091503874398767948150634765625;-0.66857072895781077814802983994013629853725433349609375;0.977761640507871288008345800335519015789031982421875;0.12210326499839997682617109830971457995474338531494140625;-0.9865396175559333347138135650311596691608428955078125;-0.0842672185283881436390629460220225155353546142578125]
      mask Display: e = 0.06;c1 = [120 150 230]/255;c2 = ([120 150 230]+0)/383;c3 = ([120 150 230]+128)/383;patch([0 1 1 0],[0 0 1 1],c1);patch([0 1 1 1-e 1-e 0+e],[0 0 1 1-e 0+e 0+e],c2);patch([0 0 1 1-e 0+e 0+e],[0 1 1 1-e 1-e 0+e],c3);plot([0 1 1 0 0],[0 0 1 1 0]);disp('weights');
  "IW{2,1}(5,:)'" : Constant  Value=[-0.434872023889841585742033203132450580596923828125;-0.6796224282174307962378634329070337116718292236328125;0.2304581629269512876856396133007365278899669647216796875;0.028292983768810502087642788637822377495467662811279296875;-0.47453388982084654390547484581475146114826202392578125;-0.45479071516655888984814737341366708278656005859375;0.0185868937412208001802582657546736299991607666015625;0.25757098223861485397634396576904691755771636962890625;-0.64637088710523948886788048184826038777828216552734375;-0.9724684294061300970923866771045140922069549560546875;-0.446051634461629931127646386812557466328144073486328125;0.6303519261942784890351276771980337798595428466796875;0.5142967769102739783448896560003049671649932861328125;0.09270519029312383751939563580890535376965999603271484375;-0.1291570940188122573744067267398349940776824951171875;-0.843519430255785351846498087979853153228759765625;0.820343490845960587876106728799641132354736328125;0.29609980260111157246427637801389209926128387451171875;0.5793105379875054250504717856529168784618377685546875;-0.2013047835772938665144238257198594510555267333984375]
      mask Display: e = 0.06;c1 = [120 150 230]/255;c2 = ([120 150 230]+0)/383;c3 = ([120 150 230]+128)/383;patch([0 1 1 0],[0 0 1 1],c1);patch([0 1 1 1-e 1-e 0+e],[0 0 1 1-e 0+e 0+e],c2);patch([0 0 1 1-e 0+e 0+e],[0 1 1 1-e 1-e 0+e],c3);plot([0 1 1 0 0],[0 0 1 1 0]);disp('weights');
  "IW{2,1}(6,:)'" : Constant  Value=[-0.2652012167416135657305176209774799644947052001953125;0.37958966482309097756342453067190945148468017578125;0.072374327422401574239074761862866580486297607421875;0.5331840353293333389927965981769375503063201904296875;0.10483256382146588503445627793553285300731658935546875;-0.653694255367164078762698409263975918292999267578125;-0.804048683221585402947084730840288102626800537109375;-0.32109060114416132503123435526504181325435638427734375;0.7786746032246576465496445962344296276569366455078125;-0.145909769456667337550470620044507086277008056640625;-0.4271763705203082128747382739675231277942657470703125;-1.1131433747827539360031323667499236762523651123046875;-0.69252177736189768353369800024665892124176025390625;-0.9832918588795862557816462867776863276958465576171875;0.345931971990886710788259961191215552389621734619140625;-0.12508512204511446075372305131168104708194732666015625;-0.74385939480324392292232005274854600429534912109375;0.04041642340052808979322662708000279963016510009765625;-0.7781525205828885294323526977677829563617706298828125;-0.3353114922875664039025878082611598074436187744140625]
      mask Display: e = 0.06;c1 = [120 150 230]/255;c2 = ([120 150 230]+0)/383;c3 = ([120 150 230]+128)/383;patch([0 1 1 0],[0 0 1 1],c1);patch([0 1 1 1-e 1-e 0+e],[0 0 1 1-e 0+e 0+e],c2);patch([0 0 1 1-e 0+e 0+e],[0 1 1 1-e 1-e 0+e],c3);plot([0 1 1 0 0],[0 0 1 1 0]);disp('weights');
  "IW{2,1}(7,:)'" : Constant  Value=[0.0076567130981626263519501662813127040863037109375;0.9140696344366119330260289643774740397930145263671875;-0.72419433771433217028601347919902764260768890380859375;-0.8001895965264147481121881355647929012775421142578125;-0.393882313847218445967968136756098829209804534912109375;0.814171646882670074774068780243396759033203125;-0.3562676961769069006180643555126152932643890380859375;0.423633152621833375395254961404134519398212432861328125;0.422219301543505676210799038017285056412220001220703125;-0.5421191347882954314485459690331481397151947021484375;0.369582226146077552630941909228567965328693389892578125;-0.251928600783765721526918923700577579438686370849609375;-0.99622409409962353610268337433808483183383941650390625;-0.132597444167428413219766980546410195529460906982421875;0.470468362431292919101366578615852631628513336181640625;-0.84041063591078246641785653991973958909511566162109375;-0.249505681033445891880973022125544957816600799560546875;0.231260384740870350572805591582437045872211456298828125;-0.48497493560545112956106095225550234317779541015625;0.115631477413919991903412665124051272869110107421875]
      mask Display: e = 0.06;c1 = [120 150 230]/255;c2 = ([120 150 230]+0)/383;c3 = ([120 150 230]+128)/383;patch([0 1 1 0],[0 0 1 1],c1);patch([0 1 1 1-e 1-e 0+e],[0 0 1 1-e 0+e 0+e],c2);patch([0 0 1 1-e 0+e 0+e],[0 1 1 1-e 1-e 0+e],c3);plot([0 1 1 0 0],[0 0 1 1 0]);disp('weights');
  "IW{2,1}(8,:)'" : Constant  Value=[0.53673827747681712718730295819113962352275848388671875;-0.5316317171125739537984600247000344097614288330078125;-0.253617160600850155560692655853927135467529296875;-0.92806288715598628247249735068180598318576812744140625;-0.2883083246233015817239220268675126135349273681640625;0.7625437328998538877300461535924114286899566650390625;-0.8546537474109274779010547717916779220104217529296875;-0.418779384267346677095389395617530681192874908447265625;0.458822416877928629386218517538509331643581390380859375;-0.936420330611999585102012133575044572353363037109375;-0.468136846042095655651138486064155586063861846923828125;0.83332307759643864386589484638534486293792724609375;0.5653454064984917426528454598155803978443145751953125;0.4174521517387095315143596963025629520416259765625;-0.25642221920146968106024587541469372808933258056640625;-0.259919083734991673839687109648366458714008331298828125;-0.311533958855341019944518166084890253841876983642578125;0.7427098419925588501655511208809912204742431640625;0.029424889122037001243370468728244304656982421875;-0.37342499333784662240987017867155373096466064453125]
      mask Display: e = 0.06;c1 = [120 150 230]/255;c2 = ([120 150 230]+0)/383;c3 = ([120 150 230]+128)/383;patch([0 1 1 0],[0 0 1 1],c1);patch([0 1 1 1-e 1-e 0+e],[0 0 1 1-e 0+e 0+e],c2);patch([0 0 1 1-e 0+e 0+e],[0 1 1 1-e 1-e 0+e],c3);plot([0 1 1 0 0],[0 0 1 1 0]);disp('weights');
  "IW{2,1}(9,:)'" : Constant  Value=[0.133894745839812145948855004462529905140399932861328125;0.251202969899141148601984241395257413387298583984375;0.662945035672104499013812528573907911777496337890625;-0.267371881262133015422222115375916473567485809326171875;0.1407441393169061860657365059523726813495159149169921875;0.01870649211412404866461400843036244623363018035888671875;-0.52817318512708055777693516574800014495849609375;0.494344731581952190335726982084452174603939056396484375;-0.84553873409395030602553333665127865970134735107421875;0.987907870625776229900338876177556812763214111328125;1.0028554160722860100207753930590115487575531005859375;0.7685372947773128071702330998959951102733612060546875;0.195225055066407138237849494544207118451595306396484375;0.42398838587524056986666209922987036406993865966796875;0.326314426863318962634963327218429185450077056884765625;0.9657350174384902175006573088467121124267578125;0.1244155713040005217795425096483086235821247100830078125;0.66776378284018722553128100116737186908721923828125;-0.5286861208721145288791376515291631221771240234375;-0.9947314935101105870529636376886628568172454833984375]
      mask Display: e = 0.06;c1 = [120 150 230]/255;c2 = ([120 150 230]+0)/383;c3 = ([120 150 230]+128)/383;patch([0 1 1 0],[0 0 1 1],c1);patch([0 1 1 1-e 1-e 0+e],[0 0 1 1-e 0+e 0+e],c2);patch([0 0 1 1-e 0+e 0+e],[0 1 1 1-e 1-e 0+e],c3);plot([0 1 1 0 0],[0 0 1 1 0]);disp('weights');
  Mux : Mux  Inputs=20
      mask Display: e = 0.06;c1 = [120 150 230]/255;c2 = ([120 150 230]+0)/383;c3 = ([120 150 230]+128)/383;patch([0 1 1 0],[0 0 1 1],c1);patch([0 1 1 1-e 1-e 0+e],[0 0 1 1-e 0+e 0+e],c2);patch([0 0 1 1-e 0+e 0+e],[0 1 1 1-e 1-e 0+e],c3);plot([0 1 1 0 0],[0 0 1 1 0]);disp('Mux');
  dotprod{1..20} (20 alike) : neural/Weight Functions/dotprod
  "lz{2,1}" : Outport
      mask Display: e = 0.06;c1 = [120 230 180]/255;c2 = ([120 230 180]+0)/(256+128);c3 = ([120 230 180]+128)/(256+128);patch([0 1 1 0],[0 0 1 1],c1);patch([0 1 1 1-e 1-e 0+e],[0 0 1 1-e 0+e 0+e],c2);patch([0 0 1 1-e 0+e 0+e],[0 1 1 1-e 1-e 0+e],c3);plot([0 1 1 0 0],[0 0 1 1 0]);
  wires:
  "IW{2,1}(1,:)'"/1 -> dotprod1/1
  "ad{2,1}"/1 -> dotprod1/2, dotprod2/2, dotprod3/2, dotprod4/2, dotprod5/2, dotprod6/2, dotprod7/2, dotprod8/2, dotprod9/2, dotprod10/2, dotprod11/2, dotprod12/2, dotprod13/2, dotprod14/2, dotprod15/2, dotprod16/2, dotprod17/2, dotprod18/2, dotprod19/2, dotprod20/2
  dotprod1/1 -> Mux/1
  "IW{2,1}(2,:)'"/1 -> dotprod2/1
  dotprod2/1 -> Mux/2
  "IW{2,1}(3,:)'"/1 -> dotprod3/1
  dotprod3/1 -> Mux/3
  "IW{2,1}(4,:)'"/1 -> dotprod4/1
  dotprod4/1 -> Mux/4
  "IW{2,1}(5,:)'"/1 -> dotprod5/1
  dotprod5/1 -> Mux/5
  "IW{2,1}(6,:)'"/1 -> dotprod6/1
  dotprod6/1 -> Mux/6
  "IW{2,1}(7,:)'"/1 -> dotprod7/1
  dotprod7/1 -> Mux/7
  "IW{2,1}(8,:)'"/1 -> dotprod8/1
  dotprod8/1 -> Mux/8
  "IW{2,1}(9,:)'"/1 -> dotprod9/1
  dotprod9/1 -> Mux/9
  "IW{2,1}(10,:)'"/1 -> dotprod10/1
  dotprod10/1 -> Mux/10
  "IW{2,1}(11,:)'"/1 -> dotprod11/1
  dotprod11/1 -> Mux/11
  "IW{2,1}(12,:)'"/1 -> dotprod12/1
  dotprod12/1 -> Mux/12
  "IW{2,1}(13,:)'"/1 -> dotprod13/1
  dotprod13/1 -> Mux/13
  "IW{2,1}(14,:)'"/1 -> dotprod14/1
  dotprod14/1 -> Mux/14
  "IW{2,1}(15,:)'"/1 -> dotprod15/1
  dotprod15/1 -> Mux/15
  "IW{2,1}(16,:)'"/1 -> dotprod16/1
  dotprod16/1 -> Mux/16
  "IW{2,1}(17,:)'"/1 -> dotprod17/1
  dotprod17/1 -> Mux/17
  "IW{2,1}(18,:)'"/1 -> dotprod18/1
  dotprod18/1 -> Mux/18
  "IW{2,1}(19,:)'"/1 -> dotprod19/1
  dotprod19/1 -> Mux/19
  "IW{2,1}(20,:)'"/1 -> dotprod20/1
  dotprod20/1 -> Mux/20
  Mux/1 -> "lz{2,1}"/1

== system nn_fuel_control_6_20/Air Fuel Control Model 1/Feed-Forward Neural Network/Layer 3/Delays 1 ==
  "p{3}" : Inport  PortDimensions=20
      mask Display: e = 0.06;c1 = [120 230 180]/255;c2 = ([120 230 180]+0)/(256+128);c3 = ([120 230 180]+128)/(256+128);patch([0 1 1 0],[0 0 1 1],c1);patch([0 1 1 1-e 1-e 0+e],[0 0 1 1-e 0+e 0+e],c2);patch([0 0 1 1-e 0+e 0+e],[0 1 1 1-e 1-e 0+e],c3);plot([0 1 1 0 0],[0 0 1 1 0]);
  mux : Mux  Inputs=1
      mask Display: e = 0.06;c1 = [120 150 230]/255;c2 = ([120 150 230]+0)/383;c3 = ([120 150 230]+128)/383;patch([0 1 1 0],[0 0 1 1],c1);patch([0 1 1 1-e 1-e 0+e],[0 0 1 1-e 0+e 0+e],c2);patch([0 0 1 1-e 0+e 0+e],[0 1 1 1-e 1-e 0+e],c3);plot([0 1 1 0 0],[0 0 1 1 0]);disp('Mux')
  "pd{3,2}" : Outport
      mask Display: e = 0.06;c1 = [120 230 180]/255;c2 = ([120 230 180]+0)/(256+128);c3 = ([120 230 180]+128)/(256+128);patch([0 1 1 0],[0 0 1 1],c1);patch([0 1 1 1-e 1-e 0+e],[0 0 1 1-e 0+e 0+e],c2);patch([0 0 1 1-e 0+e 0+e],[0 1 1 1-e 1-e 0+e],c3);plot([0 1 1 0 0],[0 0 1 1 0]);
  wires:
  "p{3}"/1 -> mux/1
  mux/1 -> "pd{3,2}"/1
